simulink model "Lab3"  (R2016b)
settings: Solver=FixedStepAuto  StartTime=0.0  StopTime=1.5  FixedStep=2e-5  RelTol=1e-5  EnableMultiTasking=on
libraries: commchan3 x1, commsink2 x1, dsparch4 x1, commrandsrc2 x1, dspsigops x1
settings Model: Creator=Dennis Silage  LastModifiedBy=avile
settings DataIOCC: LimitDataPoints=on  SaveFormat=Array  SignalLoggingSaveFormat=ModelDataLogs
settings OptimizationCC: ExpressionDepthLimit=2147483647  InitFltsAndDblsToZero=on  LifeSpan=inf
settings DebuggingCC: UnderspecifiedInitializationDetection=Classic  MergeDetectMultiDrivingBlocksExec=none  FcnCallInpInsideContextMsg=warning  StateNameClashWarn=warning  SFUnexpectedBacktrackingDiag=warning  SFNoUnconditionalDefaultTransitionDiag=warning  SFExecutionAtInitializationDiag=none
settings HardwareCC: ProdBitPerPointer=32  ProdBitPerSizeT=32  ProdBitPerPtrDiffT=32  ProdLargestAtomicFloat=None  ProdIntDivRoundTo=Undefined  ProdEndianess=Unspecified  ProdWordSize=32  ProdHWDeviceType=32-bit Generic
settings ModelReferenceCC: PropagateSignalLabelsOutOfModel=off
settings GRTTargetCC: TargetLangStandard=C89/C90 (ANSI)  GeneratePreprocessorConditionals=Disable all  CombineOutputUpdateFcns=off  GRTInterface=on
settings ConfigComp: CovMetricSettings=dw  CovHtmlReporting=on  CovSaveCumulativeToWorkspaceVar=on  CovSaveSingleToWorkspaceVar=on  CovExternalEMLEnable=off  CovSFcnEnable=off

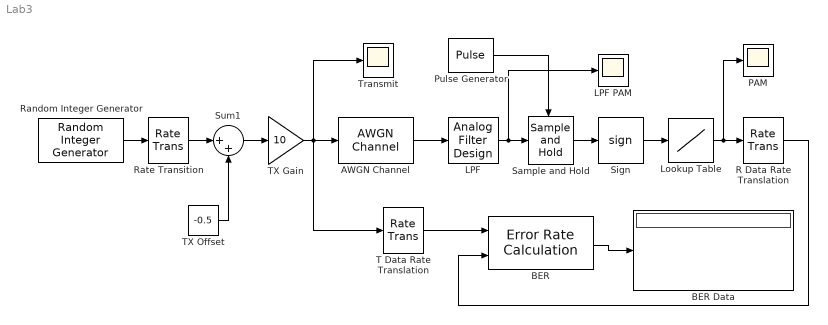
== system Lab3 ==
  AWGN Channel : commchan3/AWGN Channel  InputProcessing=Inherited (this choice will be removed - see release notes)  seed=randseed  noiseMode=Variance from mask  EbNodB=10  EsNodB=10  SNRdB=10  bitsPerSym=1  Ps=1  Tsym=1  variance=0
  BER : commsink2/Error Rate Calculation  N=2  st_delay=0  cp_mode=Entire frame  subframe=[]  PMode=Port  WsName=ErrorVec  RsMode2=off  stop=off  numErr=100  maxBits=1e6
  BER Data : Display
  LPF : dsparch4/Analog Filter Design  method=Bessel  filttype=Lowpass  N=5  Wlo=2*pi*5555  Whi=80  Rp=0.1  Rs=40
  LPF PAM : Scope
  Lookup Table : Lookup_n-D  NumberOfTableDimensions=1  BreakpointsForDimension1=[-1,0,1]  BreakpointsForDimension3=[5, 7]  Table=[-5,5,5]  InternalRulePriority=Speed  RndMeth=Simplest  InputSameDT=on
  PAM : Scope
  Pulse Generator : DiscretePulseGenerator  PulseType=Time based  Amplitude=12  Period=16e-5  PulseWidth=12.5  PhaseDelay=4e-5
  R Data Rate Translation : RateTransition  OutPortSampleTime=150e-6
  Random Integer Generator : commrandsrc2/Random Integer Generator  mul=2  seed=12  Ts=150e-6  frameBased=off  sampPerFrame=50  orient=on  outDataType=double
  Rate Transition : RateTransition  OutPortSampleTime=2e-5
  Sample and Hold : dspsigops/Sample and Hold  trig=Rising edge  initCond=0  latchinput=off
  Sign : Signum
  Sum1 : Sum  Inputs=|++
  T Data Rate Translation : RateTransition  OutPortSampleTime=150e-6
  TX Gain : Gain  Gain=10
  TX Offset : Constant  Value=-0.5
  Transmit : Scope
  wires:
  Pulse Generator/1 -> Sample and Hold/Trigger
  TX Gain/1 -> T Data Rate Translation/1, Transmit/1, AWGN Channel/1
  Sign/1 -> Lookup Table/1
  Random Integer Generator/1 -> Rate Transition/1
  Rate Transition/1 -> Sum1/1
  Sum1/1 -> TX Gain/1
  TX Offset/1 -> Sum1/2
  Sample and Hold/1 -> Sign/1
  R Data Rate Translation/1 -> BER/2
  BER/1 -> BER Data/1
  Lookup Table/1 -> R Data Rate Translation/1, PAM/1
  T Data Rate Translation/1 -> BER/1
  AWGN Channel/1 -> LPF/1
  LPF/1 -> Sample and Hold/1, LPF PAM/1
